simulink model "simple_oscillator"  (R2020a)
settings: Solver=VariableStepAuto  StartTime=0.0  StopTime=60  RelTol=1e-7
settings Model: Creator=Tomo  LastModifiedBy=Tomo

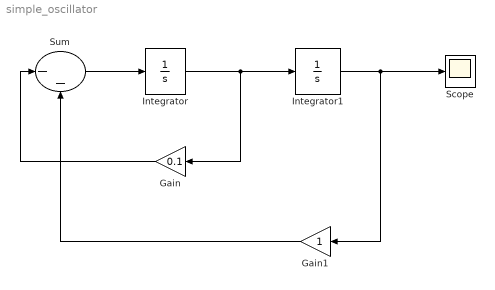
== system simple_oscillator ==
  Gain : Gain  Gain=0.1
  Gain1 : Gain
  Integrator : Integrator
  Integrator1 : Integrator  InitialCondition=1
  Scope : Scope
  Sum : Sum  Inputs=|--
  wires:
  Sum/1 -> Integrator/1
  Integrator/1 -> Gain/1, Integrator1/1
  Integrator1/1 -> Gain1/1, Scope/1
  Gain1/1 -> Sum/2
  Gain/1 -> Sum/1
